simulink model "testFliter"  (R2023b)
settings: Solver=FixedStepDiscrete  StartTime=0.0  StopTime=1/50*20  FixedStep=Ts  RelTol=1e-3
model workspace (MAT data in the model file):
  Ts = 0.0001
libraries: spspowerguiLib x1, simulink x1
settings Model: Creator=she  LastModifiedBy=she
settings DataIOCC: ReturnWorkspaceOutputs=off
settings OptimizationCC: DefaultParameterBehavior=Inlined  EnhancedBackFolding=on  PassReuseOutputArgsAs=Individual arguments  ZeroExternalMemoryAtStartup=off  ZeroInternalMemoryAtStartup=off  OptimizeBlockOrder=speed  DifferentSizesBufferReuse=on  EfficientTunableParamExpr=on
settings DebuggingCC: ParameterTunabilityLossMsg=error
settings ModelReferenceCC: EnableRefExpFcnMdlSchedulingChecks=on
settings SFSimCC: SimCustomHeaderCode="#include \"user_lib_filter.h\""  SimUserLibraries=user_lib_filter.a  MATLABDynamicMemAlloc=off
settings RTWCC: Description=Embedded Coder  SystemTargetFile=ert.tlc  TemplateMakefile=ert_default_tmf
settings CodeAppCC: ForceParamTrailComments=on  IgnoreCustomStorageClasses=off  OperatorAnnotations=on  SimulinkDataObjDesc=on  SFDataObjDesc=on  InsertBlockDesc=on
settings ERTTargetCC: TargetLangStandard=C99 (ISO)  GenerateSampleERTMain=on  InlinedParameterPlacement=NonHierarchical  ERTCustomFileTemplate=example_file_process.tlc

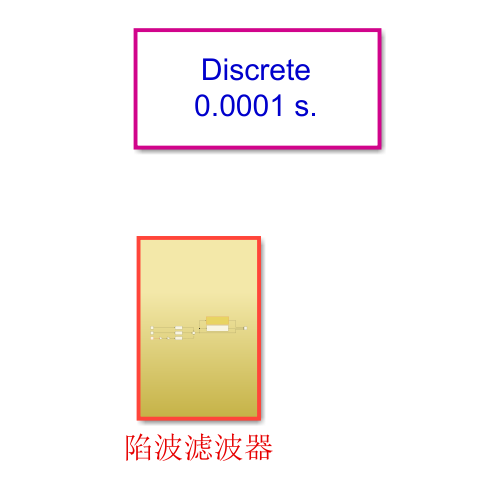
[thumbnail: Simulink's stored preview of the top-level diagram]
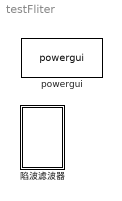
== system testFliter ==
  powergui : spspowerguiLib/powergui  Priority=1  SimulationMode=Discrete  SampleTime=Ts  frequency=60  Iterations=50  frequencyindice=60  Pbase=100e6  ErrMax=1e-4  UnitsV=kV  UnitsW=MW  buscounter=0  FunctionMessages=off  echomessages=off  EnableUseOfTLC=off  CurrentSourceSwitches=off  DisableSnubberDevices=off  DisableRonSwitches=off  DisableVfSwitches=off  DisplayEquations=off  AutomaticDiscreteSolvers=off  SolverType=Tustin/Backward Euler (TBE)  Interpol=off  ExternalGateDelay=off  methode=off  Ts=100  x0status=blocks  SPID=on  SwTol=0  HookPort=off  NonlinearTolerance=1e-4  nMaxIteration=100  ContinueOnMaxIteration=off  RestoreLinks=warning  ResistiveCurrentMeasurement=off  Frange=[0:2:500]  Ylog=off  Xlog=on  ShowGrid=off  save=off  variable=ZData  structure=0  ZoomFFT=off  StartTime=0.0  cycles=1  DisplayStyle=1  fundamental=60  FreqAxis=off  MaxFrequency=1000  frequencyindicesteady=1  RmsSteady=1  display=off
  陷波滤波器 : Subsystem

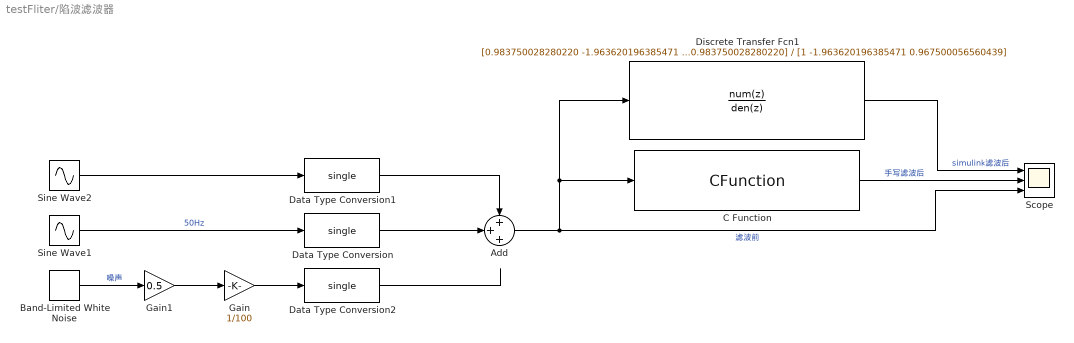
== system testFliter/陷波滤波器 ==
  Add : Sum  Inputs=+++  OutDataTypeStr=single  RndMeth=Nearest
  Band-Limited White Noise : simulink/Sources/Band-Limited White Noise  Cov=[0.1]  Ts=Ts  seed=[23341]
  C Function : CFunction  OutputCode=y=USER_LIB_FILTER_float_notchFilter_calcu(u, &test_notchFilter_str);  StartCode=USER_LIB_FILTER_void_notchFilter_init(&test_notchFilter_str,1.9,100, 1/10e3);
  Data Type Conversion : DataTypeConversion  OutDataTypeStr=single  RndMeth=Nearest  SaturateOnIntegerOverflow=off
  Data Type Conversion1 : DataTypeConversion  OutDataTypeStr=single  RndMeth=Nearest  SaturateOnIntegerOverflow=off
  Data Type Conversion2 : DataTypeConversion  OutDataTypeStr=single  RndMeth=Nearest  SaturateOnIntegerOverflow=off
  Discrete Transfer Fcn1 : DiscreteTransferFcn  Numerator=[0.983750028280220 -1.963620196385471 0.983750028280220]  Denominator=[1 -1.963620196385471 0.967500056560439]
  Gain : Gain  Gain=1/100  OutDataTypeStr=single  RndMeth=Nearest
  Gain1 : Gain  Gain=0.5  OutDataTypeStr=single  RndMeth=Nearest
  Scope : Scope  NumInputPorts=3
  Sine Wave1 : Sin  Amplitude=2  Frequency=2*pi*100  SampleTime=Ts
  Sine Wave2 : Sin  Amplitude=2  Frequency=2*pi*150  SampleTime=Ts
  wires:
  Sine Wave2/1 -> Data Type Conversion1/1
  C Function/1 -> Scope/2  "手写滤波后"
  Add/1 -> Discrete Transfer Fcn1/1, C Function/1, Scope/3  "滤波前"
  Data Type Conversion2/1 -> ?
  Data Type Conversion1/1 -> Add/1
  Band-Limited White Noise/1 -> Gain1/1  "噪声"
  Sine Wave1/1 -> Data Type Conversion/1  "50Hz"
  Gain/1 -> Data Type Conversion2/1
  Data Type Conversion/1 -> Add/2
  Gain1/1 -> Gain/1
  Discrete Transfer Fcn1/1 -> Scope/1  "simulink滤波后"
